simulink model "testf23"  (R2021b)
settings: Solver=FixedStepAuto  StartTime=0.0  StopTime=20  FixedStep=0.01  RelTol=1e-3
libraries: simulink x2
settings Model: Creator=asus  LastModifiedBy=Newsky

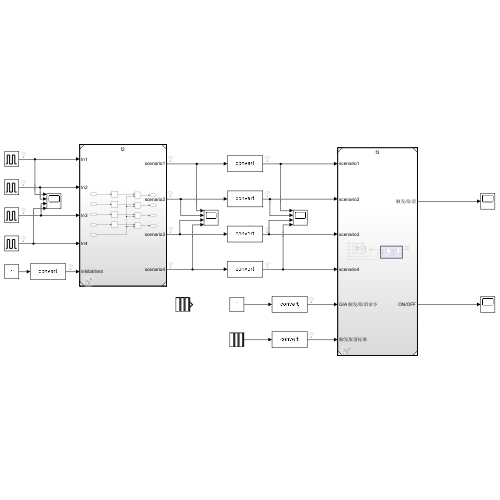
[thumbnail: Simulink's stored preview of the top-level diagram]
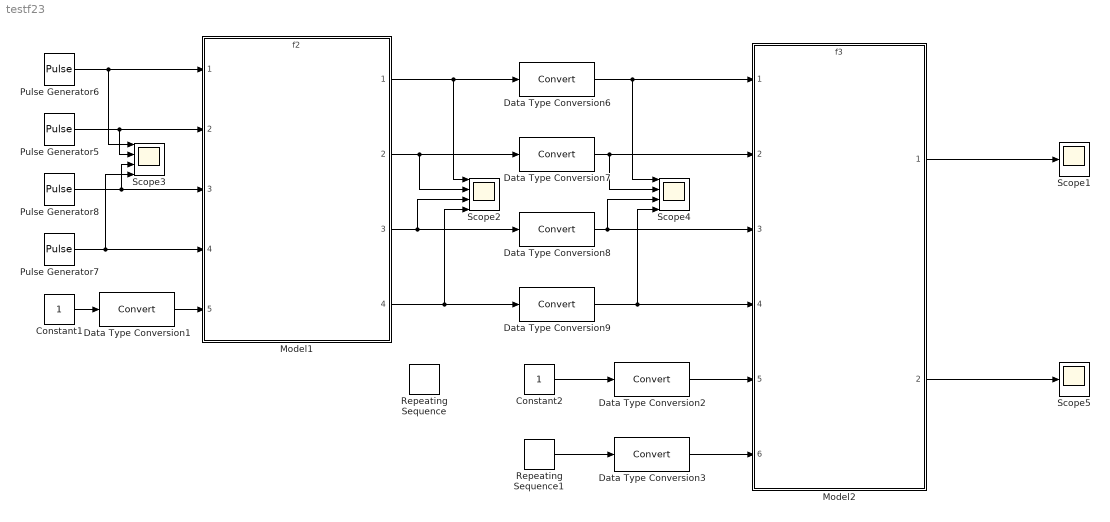
== system testf23 ==
  Constant1 : Constant
  Constant2 : Constant
  Data Type Conversion{1..3,6..9} (7 alike) : DataTypeConversion
  Model1 : ModelReference  ModelNameDialog=f2.slx  SimulationMode=Normal  ModelReferenceVersion=1.7
  Model2 : ModelReference  ModelNameDialog=f3.slx  SimulationMode=Normal  ModelReferenceVersion=1.21
  Pulse Generator5 : DiscretePulseGenerator  PulseType=Time based  Amplitude=5  Period=10  PulseWidth=50
  Pulse Generator6 : DiscretePulseGenerator  PulseType=Time based  Amplitude=2  Period=10  PulseWidth=50
  Pulse Generator7 : DiscretePulseGenerator  PulseType=Time based  Amplitude=0  Period=10  PulseWidth=50
  Pulse Generator8 : DiscretePulseGenerator  PulseType=Time based  Amplitude=5  Period=10  PulseWidth=20
  Repeating Sequence : simulink/Sources/Repeating Sequence  rep_seq_t=[0 8 8.01 10]  rep_seq_y=[1 1 0 0]
  Repeating Sequence1 : simulink/Sources/Repeating Sequence  rep_seq_t=[0 8 8.01 10]  rep_seq_y=[1 1 0 0]
  Scope1 : Scope
  Scope2 : Scope  NumInputPorts=4
  Scope3 : Scope  NumInputPorts=4
  Scope4 : Scope  NumInputPorts=4
  Scope5 : Scope
  wires:
  Pulse Generator8/1 -> Scope3/3, Model1/3
  Pulse Generator6/1 -> Scope3/1, Model1/1
  Pulse Generator5/1 -> Scope3/2, Model1/2
  Model1/3 -> Data Type Conversion8/1, Scope2/3
  Model1/1 -> Scope2/1, Data Type Conversion6/1
  Constant1/1 -> Data Type Conversion1/1
  Data Type Conversion1/1 -> Model1/5
  Pulse Generator7/1 -> Scope3/4, Model1/4
  Model1/4 -> Scope2/4, Data Type Conversion9/1
  Model1/2 -> Scope2/2, Data Type Conversion7/1
  Model2/1 -> Scope1/1
  Data Type Conversion2/1 -> Model2/5
  Data Type Conversion3/1 -> Model2/6
  Data Type Conversion7/1 -> Model2/2, Scope4/2
  Data Type Conversion9/1 -> Scope4/4, Model2/4
  Data Type Conversion6/1 -> Model2/1, Scope4/1
  Data Type Conversion8/1 -> Model2/3, Scope4/3
  Model2/2 -> Scope5/1
  Repeating Sequence1/1 -> Data Type Conversion3/1
  Constant2/1 -> Data Type Conversion2/1
